simulink model "FSM_Model"  (R2020b)
settings: Solver=VariableStepAuto  StartTime=0.0  StopTime=10.0  RelTol=1e-3
model workspace (MAT data in the model file):
  TrqICMax = 175
  TrqMGUMax = 150
  TrqMax = 325
  brkTrqMGU = 150
  brkTrqMax = 700
  fuelCapacity = 35
settings Model: Creator=mordi  LastModifiedBy=mordi

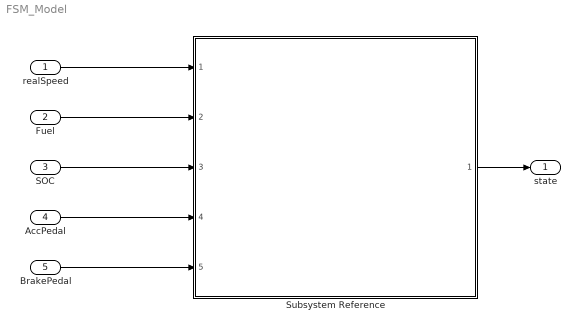
== system FSM_Model ==
  realSpeed : Inport
  Fuel : Inport  Port=2
  SOC : Inport  Port=3
  AccPedal : Inport  Port=4
  BrakePedal : Inport  Port=5
  Subsystem Reference : Subsystem  ReferencedSubsystem=stateMachine
  state : Outport
  wires:
  realSpeed/1 -> Subsystem Reference/1
  Fuel/1 -> Subsystem Reference/2
  SOC/1 -> Subsystem Reference/3
  AccPedal/1 -> Subsystem Reference/4
  BrakePedal/1 -> Subsystem Reference/5
  Subsystem Reference/1 -> state/1
